simulink model "JenaFox_Klostermair_Neuronal_Controller"  (R2020b)
settings: Solver=ode23s  StartTime=0.0  StopTime=20  MaxStep=maxStep  RelTol=relTol  AbsTol=absTol
InitFcn:
  | Fox_param;
undefined symbols (not defined in the file or in its folder): amplifier, c_coupling_hip, c_coupling_knee, c_hs, d_coupling_knee, d_hs, g, hip_i, hip_Jm, hip_k, hip_Mrg, hip_Mrhg, hip_na, hip_Ra, IC_motor_hip_l, IC_motor_hip_r, IC_motor_knee_l, IC_motor_knee_r, IC_phi_hip_l, IC_phi_hip_r, IC_v_motor_hip, IC_v_motor_knee, k_gx, k_gy, knee_i, knee_Jm, knee_k, knee_Mrg, knee_Mrhg, knee_na, knee_Ra, mu_slide, mu_stick, smiData, v_gx_max, v_gy_max, vLimit, X, Y, Z
libraries: sm_lib x38, nesl_utility x26, simulink x16, simulink_extras x8
(part 3 of 3)

== matlab function JenaFox_Klostermair_Neuronal_Controller/joint voltage calculation ==
  data: U output; phi input; v_phi input; GC input
function U = rb_control(phi,v_phi,GC)%, v_COM)

% calculates the motor torques for the runbot model (method described in Geng 2009 IEEE Trans. Mech.)
% the following indices stand for joint:
% 1 - right hip     3 - right knee
% 2 - left hip      4 - left knee


U=zeros(4,1);
phi_eq=zeros(4,1);

%% define constants

alpha=10;    %gain for equilibrium point calculation in hip joint
bbeta=0.03;  %gain for joint stiffness calculation
gamma=0.001;%base level stiffness
deltah=0.8;   %damping coefficient hip
deltak=0.07; %damping coefficient knee
phi0=-5;    %offset angle [deg]

%a_ext=phi0+2;


%% define motor neuron activity

M_eh=400;      %extensor neuron hip
M_fh=350;      %flexor neuron hip

% scale torques
ht_f=200;      %hip torque in flight
ht_s=250;       %hip torque in stance
kt_s=60;         %knee torque in stance
kt_f=800;    %knee torque in flight

%% calculate torques
K=bbeta*(M_eh+M_fh+gamma);   %21
switch GC
    case 1
        %single support left
        %right leg
        phi_eq(1)=phi0-alpha*(M_eh-M_fh)/K;         %right hip (AEA)
        U(1)=K*(phi_eq(1)-phi(1))-deltah*v_phi(1);
        if phi(1)>phi_eq(1)-1
            U(3)=K*(-90-phi(3))-deltak*v_phi(3);         %right knee bends
        else
            U(3)=K*(2-phi(3))-deltak*v_phi(3);         %right knee stays extended
        end
        %left leg
        phi_eq(2)=phi0+alpha*(M_eh-M_fh)/K;              %left hip (PEA)
        U(2)=K*(phi_eq(2)-phi(2))-deltah*v_phi(2);
        U(4)=K*(2-phi(4))-deltak*v_phi(4);          %left knee extends/stays extended
        % scale torques
        U(1)=U(1)/ht_f;
        U(3)=U(3)/kt_f;
        U(2)=U(2)/ht_s;
        U(4)=U(4)/kt_s;
    case 2
        %double support after touch down right
        %right leg
        phi_eq(1)=phi0+alpha*(M_eh-M_fh)/K;         %right hip(PEA)
        U(1)=K*(phi_eq(1)-phi(1))-deltah*v_phi(1);
        U(3)=K*(2-phi(3))-deltak*v_phi(3);       %right knee extends
        %left leg
        phi_eq(2)=phi0-alpha*(M_eh-M_fh)/K;          %left hip (AEA)
        U(2)=K*(phi_eq(2)-phi(2))-deltah*v_phi(2);
        if phi_eq(2)>phi(2)
            U(4)=K*(2-phi(4))-deltak*v_phi(4);           %left knee stays extended
        else
            U(4)=K*(-90-phi(4))-deltak*v_phi(4);           %left knee starts to flex
        end
        U(1)=U(1)/ht_s;
        U(3)=U(3)/kt_s;
        U(2)=U(2)/ht_s;
        U(4)=U(4)/kt_s;
    case 3
        %single support right leg
        %right leg
        phi_eq(1)=phi0+alpha*(M_eh-M_fh)/K;              %right hip (PEA)
        U(1)=K*(phi_eq(1)-phi(1))-deltah*v_phi(1);
        U(3)=K*(2-phi(3))-deltak*v_phi(3);          %right knee extends/stays extended
        %left leg
        phi_eq(2)=phi0-alpha*(M_eh-M_fh)/K;         %left hip (AEA)
        U(2)=K*(phi_eq(2)-phi(2))-deltah*v_phi(2);
        if phi(2)>phi_eq(2)-1
            U(4)=K*(-90-phi(4))-deltak*v_phi(4);         %left knee bends
        else
            U(4)=K*(2-phi(4))-deltak*v_phi(4);         %left knee stays extended
        end
        U(1)=U(1)/ht_s;
        U(3)=U(3)/kt_s;
        U(2)=U(2)/ht_f;
        U(4)=U(4)/kt_f;
    case 4
        %double support after touch down left
        %right leg
        phi_eq(1)=phi0-alpha*(M_eh-M_fh)/K;          %right hip (AEA)
        U(1)=K*(phi_eq(1)-phi(1))-deltah*v_phi(1);
        if phi_eq(1)>phi(1)
            U(3)=K*(2-phi(3))-deltak*v_phi(3);           %right knee stays extended
        else
            U(3)=K*(-90-phi(3))-deltak*v_phi(3);           %right knee starts to flex
        end
        %left leg
        phi_eq(2)=phi0+alpha*(M_eh-M_fh)/K;         %left hip(AEA)
        U(2)=K*(phi_eq(2)-phi(2))-deltah*v_phi(2);
        U(4)=K*(2-phi(4))-deltak*v_phi(4);       %left knee extends
        U(1)=U(1)/ht_s;
        U(3)=U(3)/kt_s;
        U(2)=U(2)/ht_s;
        U(4)=U(4)/kt_s;
end

== matlab function JenaFox_Klostermair_Neuronal_Controller/MATLAB Function ==
  settings: updateMethod=DISCRETE
  data: phi input; output_U output; GC input; t input
function output_U = NeuronalController(phi, GC, t)
    % Declare persistent variables to maintain state between function calls
    persistent y t_before;
    
    % Initialize persistent variables if they are empty
    if isempty(y)
        y = zeros(2, 4);
        t_before = 0;
    end
    
    
    % Initialize output variable
    output_U = zeros(4, 1);
    
    % Initialize weights & thresholds
    theta_eh = 5;     % Threshold for excitatory sensor neurons at the hip
    theta_fh = -10;   % Threshold for flexor sensor neurons at the hip
    theta_ek = -3;    % Threshold for excitatory sensor neurons at the knee
    theta_fk = -80;   % Threshold for flexor sensor neurons at the knee
    theta_ar = theta_fh; % Threshold for stretch receptor neurons (hip)
    theta_g = 2;      % Threshold for ground contact sensor neurons
    gm_h = 1.5;
    gm_k = 0.9 * gm_h; % Gain for knee motor neurons
    alpha = 2;        % Slope parameter for sigmoid functions
    tau = 0.01;       % Time constant for exponential decay
    w_gm = 10;        % Weight for ground contact sensor neurons
    w_am = 15;        % Weight for stretch receptor neurons
    w_sm = 30;        % Weight for joint sensor neurons
    theta_m = 1;      % Threshold for motor neurons
    s_em = 1;         % Scaling factor for excitatory motor neurons
    s_fm = -1;        % Scaling factor for flexor motor neurons
    
    % Sensor Neurons with weights
    sr_right = w_am * (1 / (1 + exp(alpha * (phi(1) - theta_ar)))); % Stretch receptor right
    sr_left =  w_am * (1 / (1 + exp(alpha * (phi(2) - theta_ar))));  % Stretch receptor left
    
    
    gc_right = w_gm * (1 / (1 + exp(alpha * (theta_g - GC(1) + GC(2))))); % Ground contact right
    gc_left = w_gm * (1 / (1 + exp(alpha * (theta_g - GC(2) + GC(1)))));  % Ground contact left
    
    % Joint sensor neurons are all connected via inhibitory synapses
    es_right_hip = -w_sm * (1 / (1 + exp(alpha * (theta_eh - phi(1))))); % Excitatory sensor right hip
    fs_right_hip = -w_sm * (1 / (1 + exp(alpha * (phi(1) - theta_fh)))); % Flexor sensor right hip

    es_left_hip = -w_sm * (1 / (1 + exp(alpha * (theta_eh - phi(2)))));  % Excitatory sensor left hip
    fs_left_hip = -w_sm * (1 / (1 + exp(alpha * (phi(2) - theta_fh))));  % Flexor sensor left hip

    es_right_knee = -w_sm * (1 / (1 + exp(alpha * (theta_ek - phi(3))))); % Excitatory sensor right knee
    fs_right_knee = -w_sm * (1 / (1 + exp(alpha * (phi(3) - theta_fk)))); % Flexor sensor right knee

    es_left_knee = -w_sm * (1 / (1 + exp(alpha * (theta_ek - phi(4)))));  % Excitatory sensor left knee
    fs_left_knee = -w_sm * (1 / (1 + exp(alpha * (phi(4) - theta_fk))));  % Flexor sensor left knee
    
    % Weighted input to motor neurons
    ro_es_rh = es_right_hip - gc_left + gc_right;                % Weighted input for excitatory right hip
    ro_fs_rh = fs_right_hip + gc_left - gc_right;                % Weighted input for flexor right hip
    
    ro_es_lh = es_left_hip + gc_left - gc_right;                 % Weighted input for excitatory left hip
    ro_fs_lh = fs_left_hip - gc_left + gc_right;                 % Weighted input for flexor left hip
    
    ro_es_rk = es_right_knee - gc_left + gc_right + sr_right;    % Weighted input for excitatory right knee
    ro_fs_rk = fs_right_knee + gc_left - gc_right - sr_right;    % Weighted input for flexor right knee
    
    ro_es_lk = es_left_knee + gc_left - gc_right + sr_left;      % Weighted input for excitatory left knee
    ro_fs_lk = fs_left_knee - gc_left + gc_right - sr_left;      % Weighted input for flexor left knee
    
    w_neurons = [ro_es_rh, ro_fs_rh; ro_es_lh, ro_fs_lh; ro_es_rk, ro_fs_rk; ro_es_lk, ro_fs_lk]';
    
    % Motor Neurons
    y = w_neurons + y .* exp(-(t - t_before) / tau); % Update neuron states
    t_before = t; % Update time
    
    motor_sigmoid = @(y) (1 / (1 + exp(alpha * (theta_m - y)))); % Motor neuron activation function
    u_m = arrayfun(motor_sigmoid, y); % Apply activation function to all neurons
    gains = [gm_h, gm_h, gm_k, gm_k]; % Gain values for motor neurons
    
    U = 3 * gains .* (s_em * u_m(1, :) + s_fm * u_m(2, :)); % Compute motor neuron outputs
    
    % Format output
    output_U(1) = U(1);
    output_U(2) = U(2);
    output_U(3) = U(3);
    output_U(4) = U(4);
end
